simulink model "VFlexP"  (R2025a)
settings: Solver=ode23tb  StartTime=0.0  StopTime=40  FixedStep=5e-5
model workspace (MAT data in the model file):
  DCop_DCBUCK : object (value not decoded)
  Grid_CCVSC_idx = [2; 3; 4; 5; 6; 7; 8; 9; 10; 11; 12]
  Grid_CCVSCs = 1
  Grid_CCVSCs_buses = 1
  Grid_CCVSCs_toM = [0 1 0 0 0 0 0 0 0 0 0 0 ... (781 elements, 71x11)]
  Grid_C_Lines = [0.1 0.1 0.1 0.1]
  Grid_Cbuses = [0.05000002 0.10000002 0.10000002 0.10000002 0.05000002]
  Grid_DC : object (value not decoded)
  Grid_DCop_DCBUCK : object (value not decoded)
  Grid_DCop_DC_PES : object (value not decoded)
  Grid_DFIGs = 1
  Grid_DFIGs_buses = 1
  Grid_DGs : string (value not decoded)
  Grid_From_buses = [1 2 4 4]
  Grid_GFls = 1
  Grid_GFls_buses = 1
  Grid_GFr_idx = [1; 2; 3]
  Grid_GFrs = 1
  Grid_GFrs_buses = 1
  Grid_GFrs_toM = [1 0 0 0 0 0 0 0 0 1 0 0 ... (15 elements, 5x3)]
  Grid_IG_idx = 1
  Grid_IGs = 1
  Grid_IGs_buses = 1
  Grid_IGs_toM = [1; 0]
  Grid_L_Lines = [0.5 0.5 0.5 0.5]
  Grid_L_Loads = [0.000959999944704 0.000156249997559 0.00154855477548]
  Grid_Lines_fromM : object (value not decoded)
  Grid_Lines_toM : object (value not decoded)
  Grid_Load_buses = [2; 3; 4]
  Grid_Load_busesDC = []
  Grid_MGES_idx = [1; 2; 3]
  Grid_MGESs = 1
  Grid_MGESs_buses = [1; 5; 3]
  Grid_MGESs_toM = [1 0 0 0 0 0 0 0 0 1 0 0 ... (15 elements, 5x3)]
  Grid_MSGs = 1
  Grid_MSGs_buses = 1
  Grid_Nbuses = 5
  Grid_PQ_gen = [3; 2; 2]
  Grid_Ploads = [1250 4000 1250]
  Grid_PloadsDC = []
  Grid_Ps_lf = [0.274439537683 0.78 0.3]
  Grid_Qloads = [0.3 0.5 0.5]
  Grid_Qs_lf = [-0.0366071562958 0.126505596722 -0.0162964024532]
  Grid_R_Lines = [0.01 0.01 0.01 0.01]
  Grid_R_Loads = [3.9999997696 1.24999998047 3.8713869387]
  Grid_R_Loads_DC = 0
  Grid_Rcf = [50000000 50000000 50000000 50000000 50000000]
  Grid_SCs = 1
  Grid_SCs_buses = 1
  Grid_SG_idx = 1
  Grid_SGs = 1
  Grid_SGs_buses = 1
  Grid_SGs_toM = [1; 0]
  Grid_To_buses = [2 3 3 5]
  Grid_VCVSC_idx = [1; 2; 3; 4; 5; 6; 7; 8; 9; 10; 11; 12]
  Grid_VCVSCs = 1
  Grid_VCVSCs_buses = [1; 2; 3; 6; 8; 9; 12; 58; 59; 60; 63; 65]
  Grid_VCVSCs_toM = [1 0 0 0 0 0 0 0 0 0 0 0 ... (852 elements, 71x12)]
  Grid_VSM_idx = [1; 2; 3]
  Grid_VSMs = 1
  Grid_VSMs_buses = 1
  Grid_VSMs_toM = [1 0 0 0 0 0 0 0 0 1 0 0 ... (15 elements, 5x3)]
  Grid_admitt_matrix = [2.15353135314-19.7953135314i  -1.9801980198+19.801980198i; -1.9801980198+19.801980198i  2.15353135314-19.7953135314i]
  Grid_admitt_matrix_noloads = [1.98686468647-19.7953135314i  -1.9801980198+19.801980198i; -1.9801980198+19.801980198i  1.98686468647-19.7953135314i]
  Grid_bus = [1; 2; 6; 7; 8]
  Grid_busDC_complexity = [1 1 1]
  Grid_busDC_complexity_PF = [2 2 2]
  Grid_bus_complexity = [1 1 1 1 1]
  Grid_bus_complexity_PF = [1 1 1 1 1]
  Grid_buses_lf = [1; 5; 3]
  Grid_conductance_matrix = [100.00000002  -100  0; -100  200.00000002  -100; 0  -100  100.00000002]
  Grid_conductance_matrix_noloads = [100.00000002  -100  0; -100  200.00000002  -100; 0  -100  100.00000002]
  Grid_fref : object (value not decoded)
  Grid_gen_static_params : mBase (value not decoded)
  Grid_iPs_lf = [3.64378984326 1.28205128205 3.33333333333]
  Grid_iQs_lf = [-27.3170631425 7.90478860943 -61.3632366329]
  Grid_iadmitt_matrix = [2.88165849328-0.0982918688642i  2.87905051706-0.123273862303i; 2.87905051706-0.123273862303i  2.88165849328-0.0982918688642i]
  Grid_iadmitt_matrix_noloads = [37.5012524798-37.4874983544i  37.4987475202-37.5125016456i; 37.4987475202-37.5125016456i  37.5012524798-37.4874983544i]
  Grid_iconductance_matrix = [16666671.4556  16666671.4489  16666671.4456; 16666671.4489  16666671.4522  16666671.4489; 16666671.4456  16666671.4489  16666671.4556]
  Grid_iconductance_matrix_noloads = [16666671.4556  16666671.4489  16666671.4456; 16666671.4489  16666671.4522  16666671.4489; 16666671.4456  16666671.4489  16666671.4556]
  Grid_init_OK_bool = 1
  Grid_intconv_PF : object (value not decoded)
  Grid_lf_op : op_report (value not decoded)
  Grid_lineDC_complexity = [1 1]
  Grid_lineDC_complexity_PF = [2 2]
  Grid_line_complexity = [1 1 1 1]
  Grid_line_complexity_PF = [3 3 3 3]
  Grid_loadDC_complexity = []
  Grid_loadDC_complexity_PF = []
  Grid_load_complexity = [3 3 3]
  Grid_load_complexity_PF = [4 4 4]
  Grid_opDC_CCVSC : object (value not decoded)
  Grid_opDC_VSM : object (value not decoded)
  Grid_opGFr : object (value not decoded)
  Grid_opVCVSC : object (value not decoded)
  Grid_op_CCVSC : object (value not decoded)
  Grid_op_IG : object (value not decoded)
  Grid_op_MGES : object (value not decoded)
  Grid_op_SG : object (value not decoded)
  Grid_op_VSM : object (value not decoded)
  Grid_shift_lines = [0 0 0 0]
  Grid_tap_lines = [1 1 1 1]
  Grid_v_buses_mod = [1 1 1 0.9837920967 1]
  LinsysParamChangeStruct : Param1 (value not decoded)
  Lline = 0.01
  Rline = 1e-05
  linsys : object (value not decoded)
symbols that are objects in the model workspace (value not decoded): Grid_DCop_DC_PES, Grid_DCop_DCBUCK, Grid_op_CCVSC, Grid_op_IG, Grid_op_MGES, Grid_op_SG, Grid_op_VSM, Grid_opDC_CCVSC, Grid_opDC_VSM, Grid_opGFr, Grid_opVCVSC
undefined symbols (not defined in the file): block_buses_DC, block_idx, CCVSC_idx, Cf, costs, costs2, D, DFIGs_nodes, DiscIntNeverNeededParam, entity, Fb, Fi, From_nodes, grid_linsys, Grid_op_DFIG, Grid_op_DFIG_PQ, Grid_op_MSG, Grid_op_SC, Grid_op_VCVSC, H, initial_states_grid, K_1, K_3, K_5, K_A, K_C, K_IM, K_IR, K_P, K_PM, K_PR, K_S1, K_S2, K_S3, Ki_w, Kic, Kiv, Kp_id, Kp_theta, Kp_w, Kpc, Kpv, last_send, Lc, Lf, Lfd, Lkd1, Lkd2, Lkq1, Lkq2, Lkq3, Lmd, Lmq, Lsd, Lsq, m, M, Matrix_flux_to_i, mp, MSGs_buses ... (+44)
libraries: simulink x1048, eeGeneralControl x12
(part 12 of 50)

== system VFlexP/Grid/Generators/VSM/PC ==
  ioq : Inport
  iodi : Inport  Port=2
  Eref : Inport  Port=3
  vodi : Inport  Port=4
  voq : Inport  Port=5
  omegasp : Inport  Port=6
  Psp : Inport  Port=7
  Divide : Product  Inputs=*/
  Gain : Gain  Gain=1./Rv
  Gain1 : Gain  Gain=Dv
  Gain2 : Gain  Gain=1./(2*Hv)
  Integrator : Integrator  InitialCondition=Grid_op_VSM.op.States(3).x'
  Integrator1 : Integrator  InitialCondition=Grid_op_VSM.op.States(4).x'
  LPF_P : Subsystem
  LPF_Q : Subsystem
  P : InitialCondition  Commented=through
  Product{,1..3} (4 alike) : Product
  Q : InitialCondition  Commented=through
  Sum : Sum  Inputs=|++
  Sum1 : Sum  Inputs=|-+
  Sum2 : Sum  Inputs=|++
  Sum3 : Sum  Inputs=|-+
  Sum4 : Sum  Inputs=+|+|+
  Sum5 : Sum  Inputs=+-|
  Sum6 : Sum  Inputs=|+-
  Sum7 : Sum  Inputs=|+-
  Turbine model : Subsystem
  WOF_d : Subsystem  Commented=through
  Zero : Constant  Value=0  OutDataTypeStr=Inherit: Inherit via back propagation
  nq1 : Gain  Gain=nq
  omega : Outport
  Out2 : Outport  Port=2
  P_f : Outport  Port=3
  Q_f : Outport  Port=4
  wires:
  ioq/1 -> Product1/2, Product2/2  "ioq"
  iodi/1 -> Product/2, Product3/2  "iod"
  voq/1 -> Product3/1, Product1/1  "voq"
  Sum1/1 -> Q/1
  Sum/1 -> P/1
  LPF_Q/1(Q_f) -> nq1/1, Q_f/1
  LPF_P/1(P_f) -> P_f/1, Sum6/2
  Sum3/1 -> Out2/1  "vodref"
  Eref/1 -> Sum3/2  "Eref"
  nq1/1 -> Sum3/1  "nqQ"
  Product3/1 -> Sum1/2
  Product2/1 -> Sum1/1
  Product1/1 -> Sum/2
  Product/1 -> Sum/1
  vodi/1 -> Product/1, Product2/1  "vod"
  P/1 -> LPF_P/1(P)
  Q/1 -> LPF_Q/1(Q)
  omegasp/1 -> Sum5/1
  Sum5/1 -> Gain/1
  Sum4/1 -> Turbine model/1(In1)
  Sum7/1 -> Gain2/1
  Gain2/1 -> Integrator/1
  Integrator/1 -> WOF_d/1(In1), Sum2/1
  Zero/1 -> Sum2/2
  WOF_d/1(Out1) -> Gain1/1
  Gain1/1 -> Sum7/2
  Psp/1 -> Sum4/2
  Turbine model/1(Out1) -> Sum6/1
  Sum6/1 -> Divide/1
  Divide/1 -> Sum7/1
  Sum2/1 -> omega/1, Sum5/2, Divide/2
  Integrator1/1 -> Sum4/3
  Gain/1 -> Sum4/1

== system VFlexP/Grid/Generators/VSM/PI ==
  In1 : Inport
  Gain : Gain  Gain=0.1
  Gain1 : Gain  Gain=0.2
  I : Integrator  InitialCondition=Grid_op_VSM.op.States(7).x'
  Sum10 : Sum  Inputs=|++
  Out1 : Outport
  wires:
  In1/1 -> Gain1/1, Gain/1
  Sum10/1 -> Out1/1
  Gain/1 -> Sum10/1
  I/1 -> Sum10/2
  Gain1/1 -> I/1

== system VFlexP/Grid/Generators/VSM/PI1 ==
  In1 : Inport
  Gain : Gain  Gain=0.1/100/pi
  Gain1 : Gain  Gain=0.2/100/pi
  I : Integrator  InitialCondition=Grid_op_VSM.op.States(8).x'
  Sum10 : Sum  Inputs=|++
  Out1 : Outport
  wires:
  Gain1/1 -> I/1
  I/1 -> Sum10/2
  Gain/1 -> Sum10/1
  Sum10/1 -> Out1/1
  In1/1 -> Gain/1, Gain1/1

== system VFlexP/Grid/Generators/VSM/RL out ==
  note: 1) Add Subsystem or Model blocks as valid variant choices.
      | 2) You cannot connect blocks at this level. At simulation, connectivity is automatically
      | determined, based on the active variant and port name matching.
  v_in_d : Inport
  v_out_d : Inport  Port=2
  v_in_q : Inport  Port=3
  v_out_q : Inport  Port=4
  dynamic : Subsystem  VariantControl=dynamic
  static : Subsystem  VariantControl=static
  static_omega : Subsystem  VariantControl=static_omega
  id : Outport
  iq : Outport  Port=2
  v_outd : Outport  Port=3
  v_outq : Outport  Port=4

== system VFlexP/Grid/Generators/VSM/Reference frame transform1 ==
  in_d : Inport
  theta : Inport  Port=2
  in_q : Inport  Port=3
  Complex to Real-Imag : ComplexToRealImag
  Cos : Trigonometry  SCDEnableBlockLinearizationSpecification=on  Operator=cos
  Product : Product
  Real-Imag to Complex : RealImagToComplex
  Real-Imag to Complex1 : RealImagToComplex
  Sin : Trigonometry  SCDEnableBlockLinearizationSpecification=on
  out_d : Outport
  out_q : Outport  Port=2
  wires:
  in_d/1 -> Real-Imag to Complex/1
  in_q/1 -> Real-Imag to Complex/2
  Complex to Real-Imag/1 -> out_d/1
  Sin/1 -> Real-Imag to Complex1/2
  Cos/1 -> Real-Imag to Complex1/1
  theta/1 -> Cos/1, Sin/1
  Product/1 -> Complex to Real-Imag/1
  Real-Imag to Complex/1 -> Product/2
  Real-Imag to Complex1/1 -> Product/1
  Complex to Real-Imag/2 -> out_q/1

== system VFlexP/Grid/Generators/VSM/Reference frame transform2 ==
  in_d : Inport
  theta : Inport  Port=2
  in_q : Inport  Port=3
  Complex to Real-Imag : ComplexToRealImag
  Cos : Trigonometry  SCDEnableBlockLinearizationSpecification=on  Operator=cos
  Product : Product
  Real-Imag to Complex : RealImagToComplex
  Real-Imag to Complex1 : RealImagToComplex
  Sin : Trigonometry  SCDEnableBlockLinearizationSpecification=on
  out_d : Outport
  out_q : Outport  Port=2
  wires:
  Complex to Real-Imag/2 -> out_q/1
  Real-Imag to Complex1/1 -> Product/1
  Real-Imag to Complex/1 -> Product/2
  Product/1 -> Complex to Real-Imag/1
  theta/1 -> Sin/1, Cos/1
  Cos/1 -> Real-Imag to Complex1/1
  Sin/1 -> Real-Imag to Complex1/2
  Complex to Real-Imag/1 -> out_d/1
  in_q/1 -> Real-Imag to Complex/2
  in_d/1 -> Real-Imag to Complex/1

== system VFlexP/Grid/Generators/VSM/Reference frame transform3 ==
  in_d : Inport
  theta : Inport  Port=2
  in_q : Inport  Port=3
  Complex to Real-Imag : ComplexToRealImag
  Cos : Trigonometry  SCDEnableBlockLinearizationSpecification=on  Operator=cos
  Product : Product
  Real-Imag to Complex : RealImagToComplex
  Real-Imag to Complex1 : RealImagToComplex
  Sin : Trigonometry  SCDEnableBlockLinearizationSpecification=on
  out_d : Outport
  out_q : Outport  Port=2
  wires:
  in_d/1 -> Real-Imag to Complex/1
  in_q/1 -> Real-Imag to Complex/2
  Complex to Real-Imag/1 -> out_d/1
  Sin/1 -> Real-Imag to Complex1/2
  Cos/1 -> Real-Imag to Complex1/1
  theta/1 -> Sin/1, Cos/1
  Product/1 -> Complex to Real-Imag/1
  Real-Imag to Complex/1 -> Product/2
  Real-Imag to Complex1/1 -> Product/1
  Complex to Real-Imag/2 -> out_q/1

== system VFlexP/Grid/Generators/VSM/VCC ==
  note: 1) Add Subsystem or Model blocks as valid variant choices.
      | 2) You cannot connect blocks at this level. At simulation, connectivity is automatically
      | determined, based on the active variant and port name matching.
  vodref : Inport
  voqref : Inport  Port=2
  iod : Inport  Port=3
  ioq : Inport  Port=4
  omega : Inport  Port=5
  dynamic : Subsystem  VariantControl=dynamic
  dynamic_VC : Subsystem  VariantControl=dynamic_VC
  dynamic_limiting : Subsystem  VariantControl=dynamic_limiting
  static : Subsystem  VariantControl=static
  vidref : Outport
  viqref : Outport  Port=2

== system VFlexP/Grid/Generators/VSM/VI ==
  id : Inport
  iq : Inport  Port=2
  omega : Inport  Port=3
  Gain : Gain  Gain=L
  Gain1 : Gain  Gain=R
  Gain2 : Gain  Gain=L
  Gain3 : Gain  Gain=R
  Product : Product
  Product1 : Product
  Sum : Sum  Inputs=-+|
  Sum1 : Sum  Inputs=|--
  WOF_d : Subsystem  Commented=through
  WOF_q : Subsystem  Commented=through
  vd : Outport
  vq : Outport  Port=2
  wires:
  Gain/1 -> Product/1
  omega/1 -> Product/2, Product1/1
  iq/1 -> WOF_q/1(In1)
  Product/1 -> Sum/2
  id/1 -> WOF_d/1(In1)
  Gain2/1 -> Product1/2
  Product1/1 -> Sum1/1
  Gain1/1 -> Sum/1
  Gain3/1 -> Sum1/2
  Sum/1 -> vd/1
  Sum1/1 -> vq/1
  WOF_d/1(Out1) -> Gain2/1, Gain1/1
  WOF_q/1(Out1) -> Gain3/1, Gain/1

== system VFlexP/Grid/Generators/VSM/connect ==
  id : Inport
  iq : Inport  Port=2
  connect : Inport  Port=3
  Switch : Switch  Criteria=u2 > Threshold  ZeroCross=off  SaturateOnIntegerOverflow=off  InputSameDT=off
  Switch1 : Switch  Criteria=u2 > Threshold  ZeroCross=off  SaturateOnIntegerOverflow=off  InputSameDT=off
  Zero1 : Constant  Value=0  VectorParams1D=off  OutDataTypeStr=Inherit: Inherit via back propagation
  Zero2 : Constant  Value=0  VectorParams1D=off  OutDataTypeStr=Inherit: Inherit via back propagation
  id_real : Outport
  iq_real : Outport  Port=2
  connected : Outport  Port=3  OutDataTypeStr=boolean
  wires:
  Zero2/1 -> Switch1/3
  iq/1 -> Switch1/1
  Switch1/1 -> iq_real/1
  connect/1 -> Switch/2, Switch1/2, connected/1
  id/1 -> Switch/1
  Zero1/1 -> Switch/3
  Switch/1 -> id_real/1

== system VFlexP/Grid/Generators/VSM/trim_output ==
  id : Inport
  iq : Inport  Port=2
  vd : Inport  Port=3
  vq : Inport  Port=4
  Out1 : Outport
  Out2 : Outport  Port=2
  Out3 : Outport  Port=3
  Out4 : Outport  Port=4
  wires:
  iq/1 -> Out2/1
  vd/1 -> Out3/1
  vq/1 -> Out4/1
  id/1 -> Out1/1

== system VFlexP/Grid/Generators_DC/DC_PES/WOF_d ==
  In1 : Inport
  Gain : Gain  Gain=100
  Gain1 : Gain  Gain=100
  I : Integrator  InitialConditionSource=external  InitialCondition=Grid_DCop_DC_PES.op.States(4).x'
  Sum : Sum  Inputs=+-|
  Sum4 : Sum  Inputs=|+-
  Out1 : Outport
  wires:
  Sum/1 -> Out1/1
  I/1 -> Sum4/2, Sum/2
  In1/1 -> Gain1/1
  Sum4/1 -> Gain/1
  Gain/1 -> I/1
  Gain1/1 -> I/2, Sum4/1, Sum/1

== system VFlexP/Grid/Grid/Dynamic/Buses ==
  i_in : Inport
  i_out : Inport  Port=2
  Sum : Sum  Inputs=|++++
  dynamic : Subsystem  VariantControl=dynamic
  only R : Subsystem  Commented=on  VariantControl=only R
  static : Subsystem  Commented=on  VariantControl=static
  static omega : Subsystem  Commented=on  VariantControl=static omega
  v : Outport
  wires:
  static omega/1(v) -> Sum/3
  i_out/1 -> only R/2(i_out), static omega/2(i_out), static/2(i_out), dynamic/2(i_out)
  dynamic/1(v) -> Sum/1
  i_in/1 -> only R/1(i_in), static omega/1(i_in), static/1(i_in), dynamic/1(i_in)
  only R/1(v) -> Sum/4
  static/1(v) -> Sum/2
  Sum/1 -> v/1

== system VFlexP/Grid/Grid/Dynamic/Lines ==
  v_in : Inport
  v_out : Inport  Port=2
  connected : Inport  Port=3
  Constant1 : Constant  Value=zeros(1, length(R_Lines))  VectorParams1D=off
  Matrix Concatenate : Concatenate  NumInputs=3  Mode=Multidimensional array
  Selector : Selector  NumberOfDimensions=2  InputPortWidth=3  IndexOptions=Index vector (dialog),Select all  Indices=1,1  OutputSizes=1,1
  Selector1 : Selector  NumberOfDimensions=2  InputPortWidth=3  IndexOptions=Index vector (dialog),Select all  Indices=2,1  OutputSizes=1,1
  Sum : Sum  Inputs=|+++
  dynamic : Subsystem  VariantControl=dynamic
  static : Subsystem  Commented=on  VariantControl=static
  static omega : Subsystem  Commented=on  VariantControl=static_omega
  tap transformer : Subsystem
  i : Outport
  wires:
  connected/1 -> static omega/3(connected), static/3(connected), dynamic/3(connected)
  v_out/1 -> static omega/2(v_out), static/2(v_out_d), dynamic/2(v_out)
  Matrix Concatenate/1 -> dynamic/1(v_in_d), static omega/1(v_in_d), static/1(v_in)
  dynamic/1(i) -> Sum/1
  static/1(i) -> Sum/2
  static omega/1(i) -> Sum/3
  Sum/1 -> i/1
  v_in/1 -> Selector1/1, Selector/1
  Selector/1 -> tap transformer/1(in_d)
  Selector1/1 -> tap transformer/2(in_q)
  Constant1/1 -> Matrix Concatenate/3
  tap transformer/1(out_d) -> Matrix Concatenate/1
  tap transformer/2(out_q) -> Matrix Concatenate/2

== system VFlexP/Grid/Grid/Dynamic/Lines to buses ==
  i : Inport
  Complex to Real-Imag : ComplexToRealImag
  Constant1 : Constant  Value=zeros(1, length(R_Lines))  VectorParams1D=off
  Gain : Gain  Gain=1./tap_lines.*(cos(shift_lines)-1i*sin(shift_lines))
  Lines_toM : Subsystem  TreatAsAtomicUnit=on
  Matrix Concatenate : Concatenate  NumInputs=3  Mode=Multidimensional array
  Real-Imag to Complex : RealImagToComplex
  Selector : Selector  NumberOfDimensions=2  InputPortWidth=3  IndexOptions=Index vector (dialog),Select all  Indices=1,1  OutputSizes=1,1
  Selector1 : Selector  NumberOfDimensions=2  InputPortWidth=3  IndexOptions=Index vector (dialog),Select all  Indices=2,1  OutputSizes=1,1
  i_in_buses : Outport
  i_out_buses : Outport  Port=2
  wires:
  Lines_toM/2(i_to_lines) -> i_out_buses/1
  i/1 -> Lines_toM/1(i_to), Selector1/1, Selector/1
  Lines_toM/1(i_from_lines) -> i_in_buses/1
  Matrix Concatenate/1 -> Lines_toM/2(i_from)
  Real-Imag to Complex/1 -> Gain/1
  Selector1/1 -> Real-Imag to Complex/2
  Selector/1 -> Real-Imag to Complex/1
  Complex to Real-Imag/1 -> Matrix Concatenate/1
  Complex to Real-Imag/2 -> Matrix Concatenate/2
  Gain/1 -> Complex to Real-Imag/1
  Constant1/1 -> Matrix Concatenate/3

== system VFlexP/Grid/Grid/Dynamic/Loads ==
  v_in : Inport
  connected : Inport  Port=2
  iP : Inport  Port=3
  PQ : Subsystem  Commented=on  VariantControl=PQ
  Sum : Sum  Inputs=|++++++++
  dynamic PQ : Subsystem  Commented=on  VariantControl=dynamic_PQ
  parallel RL dynamic : Subsystem  Commented=on  VariantControl=dynamic
  parallel RL static : Subsystem  Commented=on  VariantControl=dynamic
  parallel RL static omega : Subsystem  Commented=on  VariantControl=dynamic
  series RL dynamic : Subsystem  Commented=on  VariantControl=dynamic
  series RL static : Subsystem  Commented=on  VariantControl=static
  series RL static omega : Subsystem  VariantControl=static_omega
  i : Outport
  wires:
  v_in/1 -> series RL dynamic/1(v_in), parallel RL dynamic/1(v_in), parallel RL static omega/1(v_in), parallel RL static/1(v_in), dynamic PQ/1(v_in), PQ/1(v_in), series RL static omega/1(v_in), series RL static/2(v_in)
  series RL dynamic/1(i) -> Sum/1
  connected/1 -> series RL dynamic/2(connected), parallel RL dynamic/2(connected), parallel RL static omega/2(connected), parallel RL static/2(connected), dynamic PQ/2(connected), PQ/2(connected), series RL static omega/2(connected), series RL static/1(connected)
  iP/1 -> PQ/3(iP), dynamic PQ/3(iP)
  series RL static/1(i) -> Sum/2
  PQ/1(i) -> Sum/4
  dynamic PQ/1(i) -> Sum/5
  series RL static omega/1(i) -> Sum/3
  Sum/1 -> i/1
  parallel RL dynamic/1(i) -> Sum/6
  parallel RL static/1(i) -> Sum/7
  parallel RL static omega/1(i) -> Sum/8

== system VFlexP/Grid/Grid/Dynamic/Loads to buses ==
  i_loads : Inport
  LoadsM : Subsystem  TreatAsAtomicUnit=on
  i_out_buses : Outport
  wires:
  i_loads/1 -> LoadsM/1(i)
  LoadsM/1(Out1) -> i_out_buses/1

== system VFlexP/Grid/Grid/Dynamic/connect ==
  note: in which load?
      | By default, the max(P)
  Assignment : Assignment  DiagnosticForDimensions=Warning  IndexOptions=Index vector (dialog)  Indices=1  OutputSizes=1
  One3 : Constant  Value=ones(1, length(L_Loads))  VectorParams1D=off  OutDataTypeStr=Inherit: Inherit via back propagation
  Step : Step  Before=1  SampleTime=0
  Out1 : Outport
  wires:
  Assignment/1 -> Out1/1
  One3/1 -> Assignment/1
  Step/1 -> Assignment/2

== system VFlexP/Grid/Grid/Dynamic/iCbuses ==
  In1 : Inport
  Constant : Constant  Value=Cbuses  VectorParams1D=off
  Constant1 : Constant  Value=C_Lines  VectorParams1D=off
  Gain : Gain  Gain=1/2
  Saturation : Saturate  UpperLimit=inf  LowerLimit=1e-3
  Subsystem : Subsystem
  Sum3 : Sum  Inputs=|-+
  Switch : Switch  Criteria=u2 > Threshold  SaturateOnIntegerOverflow=off  InputSameDT=off
  Zero : Constant  Value=zeros(1, length(From_buses))  VectorParams1D=off  OutDataTypeStr=Inherit: Inherit via back propagation
  Out1 : Outport
  wires:
  Switch/1 -> Gain/1
  Sum3/1 -> Saturation/1
  Zero/1 -> Switch/1
  Saturation/1 -> Out1/1
  Constant/1 -> Sum3/2
  Gain/1 -> Subsystem/1(In1)
  Constant1/1 -> Switch/3
  In1/1 -> Switch/2
  Subsystem/1(Out1) -> Sum3/1

== system VFlexP/Grid/Grid/Dynamic/iP ==
  note: in which load?
      | By default, the max(P)
  Assignment : Assignment  DiagnosticForDimensions=Warning  IndexOptions=Index vector (dialog)  Indices=find(Ploads == max(Ploads), 1)  OutputSizes=1
  Gain : Gain  Gain=0
  One3 : Constant  Value=zeros(1, length(L_Loads))  VectorParams1D=off  OutDataTypeStr=Inherit: Inherit via back propagation
  iP in % : Step  After=0.1  SampleTime=0  VectorParams1D=off  ZeroCross=off
  Out1 : Outport
  wires:
  One3/1 -> Assignment/1
  iP in %/1 -> Gain/1
  Assignment/1 -> Out1/1
  Gain/1 -> Assignment/2

== system VFlexP/Grid/Grid_DC/dynamic/BusesDC ==
  Input : Inport
  Input1 : Inport  Port=2
  Sum : Sum
  dynamic : Subsystem
  static : Subsystem  Commented=on
  v : Outport
  wires:
  Input/1 -> static/1(i_in), dynamic/1(i_in)
  Input1/1 -> static/2(i_out), dynamic/2(i_out)
  dynamic/1(v) -> Sum/1
  static/1(v) -> Sum/2
  Sum/1 -> v/1

== system VFlexP/Grid/Grid_DC/dynamic/DC_Lines_toM1 ==
  i : Inport
  State-Space : StateSpace  A=[]  B=[]  C=[]  D=DC.Lines_toM  InitialCondition=0  ParameterTunability=Optimized
  State-Space1 : StateSpace  A=[]  B=[]  C=[]  D=DC.Lines_fromM  InitialCondition=0  ParameterTunability=Optimized
  Transpose{,1..3} (4 alike) : Math  Operator=transpose
  i_from_lines : Outport
  i_to_lines : Outport  Port=2
  wires:
  Transpose2/1 -> State-Space1/1
  i/1 -> Transpose2/1, Transpose/1
  Transpose3/1 -> i_to_lines/1
  Transpose/1 -> State-Space/1
  State-Space1/1 -> Transpose3/1
  State-Space/1 -> Transpose1/1
  Transpose1/1 -> i_from_lines/1

== system VFlexP/Grid/Grid_DC/dynamic/DClines ==
  V_dc_In : Inport
  V_dc_out : Inport  Port=2
  Dynamic : Subsystem
  Static : Subsystem  Commented=on
  Sum4 : Sum
  i : Outport
  wires:
  V_dc_In/1 -> Static/1(V_dc_In), Dynamic/1(V_dc_In)
  V_dc_out/1 -> Dynamic/2(V_dc_Out), Static/2(V_dc_Out)
  Dynamic/1(i) -> Sum4/1
  Static/1(i) -> Sum4/2
  Sum4/1 -> i/1

== system VFlexP/Grid/Grid_DC/dynamic/Loads ==
  v_in : Inport
  connected : Inport  Port=2
  ConstI : Subsystem  Commented=on
  ConstP : Subsystem  Commented=on
  ConstR : Subsystem  Commented=on
  DynamicP : Subsystem  Commented=on
  Sum4 : Sum  Inputs=++++
  i : Outport
  wires:
  ConstR/1(i) -> Sum4/2
  ConstP/1(i) -> Sum4/1
  connected/1 -> DynamicP/2(connected), ConstI/1(connected), ConstR/2(connected), ConstP/2(connected)
  v_in/1 -> DynamicP/1(v_in), ConstR/1(v_in), ConstP/1(v_in)
  Sum4/1 -> i/1
  ConstI/1(i) -> Sum4/3
  DynamicP/1(i) -> Sum4/4

== system VFlexP/Grid/Grid_DC/dynamic/Loads to buses ==
  i_loads : Inport
  LoadsM : Subsystem  TreatAsAtomicUnit=on
  i_out_buses : Outport
  wires:
  i_loads/1 -> LoadsM/1(i)
  LoadsM/1(i_out_buses) -> i_out_buses/1

== system VFlexP/Grid/Grid_DC/static/LPF_d1 ==
  In1 : Inport
  Gain : Gain  Gain=1000
  I : Integrator  InitialCondition=DC.v
  Sum4 : Sum  Inputs=|+-
  v_buses_dc : Outport
  wires:
  Sum4/1 -> Gain/1
  In1/1 -> Sum4/1
  I/1 -> v_buses_dc/1, Sum4/2
  Gain/1 -> I/1
